simulink model "truxal_"  (R2020b)
settings: Solver=VariableStepAuto  StartTime=0.0  StopTime=5  RelTol=1e-3
settings Model: Creator=cmparedes  LastModifiedBy=Acer
settings SFSimCC: CustomCodeUndefinedFunction=UseInterfaceOnly

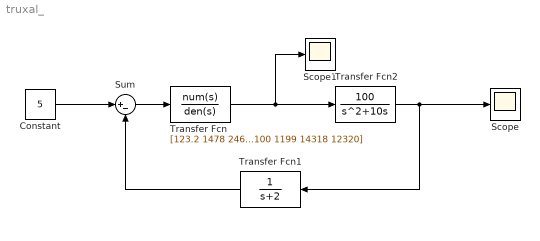
== system truxal_ ==
  Constant : Constant  Value=5
  Scope : Scope
  Scope1 : Scope
  Sum : Sum  Inputs=|+-
  Transfer Fcn : TransferFcn  Numerator=[123.2 1478 2464 0]  Denominator=[100 1199 14318 12320]
  Transfer Fcn1 : TransferFcn  Denominator=[1 2]
  Transfer Fcn2 : TransferFcn  Numerator=[100]  Denominator=[1 10 0]
  wires:
  Sum/1 -> Transfer Fcn/1
  Transfer Fcn/1 -> Scope1/1, Transfer Fcn2/1
  Transfer Fcn2/1 -> Scope/1, Transfer Fcn1/1
  Transfer Fcn1/1 -> Sum/2
  Constant/1 -> Sum/1
